simulink model "Ejercicio_2b"  (R2013a)
settings: Solver=ode45  StartTime=0.0  StopTime=40.0  RelTol=1e-3
InitFcn:
  | G1n=1;
  | G2n=1;
  | G3n=1;
  | G4n=1;
  | G5n=5;
  | G6n=1;
  | G7n=3;
  | G8n=1;
  | G1d=[1 7];
  | G2d=[1 2 3];
  | G3d=[1 4];
  | G4d=[1 0];
  | G5d=[1 7];
  | G6d=[1 5 10];
  | G7d=[1 2];
  | G8d=[1 6];
StartFcn:
  | G1n=1;
  | G2n=1;
  | G3n=1;
  | G4n=1;
  | G5n=5;
  | G6n=1;
  | G7n=3;
  | G8n=1;
  | G1d=[1 7];
  | G2d=[1 2 3];
  | G3d=[1 4];
  | G4d=[1 0];
  | G5d=[1 7];
  | G6d=[1 5 10];
  | G7d=[1 2];
  | G8d=[1 6];
settings Model: Creator=LuisFernando  LastModifiedBy=LuisFernando

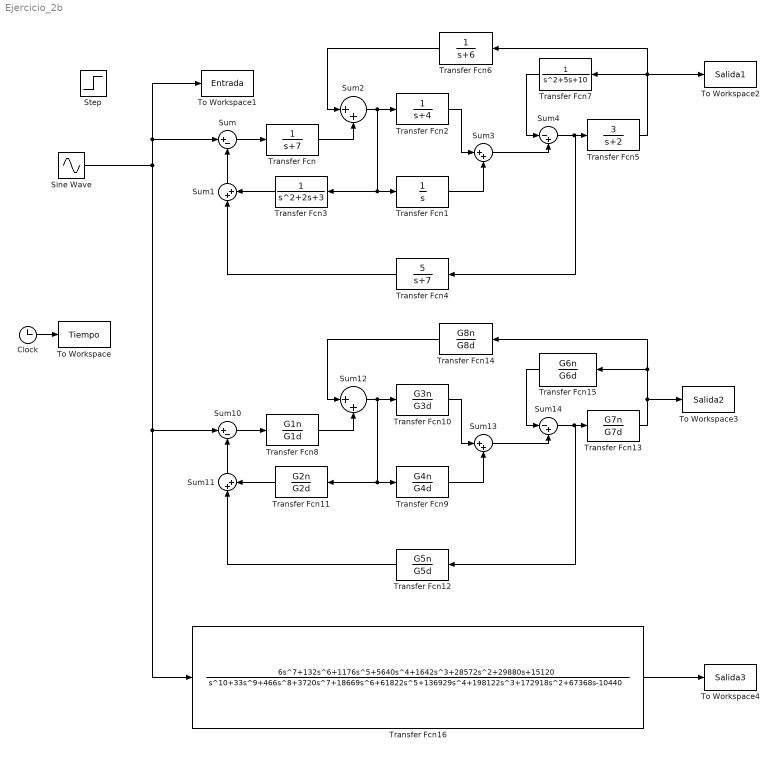
== system Ejercicio_2b ==
  Clock : Clock
  Sine Wave : Sin  Frequency=15  SampleTime=0
  Step : Step  SampleTime=0
  Sum : Sum  Inputs=|+-
  Sum{1..3,11..13} (6 alike) : Sum  Inputs=|++
  Sum10 : Sum  Inputs=|+-
  Sum14 : Sum  Inputs=|-+
  Sum4 : Sum  Inputs=|-+
  To Workspace : ToWorkspace  VariableName=Tiempo  SampleTime=-1
  To Workspace1 : ToWorkspace  VariableName=Entrada  SampleTime=-1
  To Workspace2 : ToWorkspace  VariableName=Salida1  SampleTime=-1
  To Workspace3 : ToWorkspace  VariableName=Salida2  SampleTime=-1
  To Workspace4 : ToWorkspace  VariableName=Salida3  SampleTime=-1
  Transfer Fcn : TransferFcn  Denominator=[1 7]
  Transfer Fcn1 : TransferFcn  Denominator=[1 0]
  Transfer Fcn10 : TransferFcn  Numerator=G3n  Denominator=G3d
  Transfer Fcn11 : TransferFcn  Numerator=G2n  Denominator=G2d
  Transfer Fcn12 : TransferFcn  Numerator=G5n  Denominator=G5d
  Transfer Fcn13 : TransferFcn  Numerator=G7n  Denominator=G7d
  Transfer Fcn14 : TransferFcn  Numerator=G8n  Denominator=G8d
  Transfer Fcn15 : TransferFcn  Numerator=G6n  Denominator=G6d
  Transfer Fcn16 : TransferFcn  Numerator=[6,132,1176,5640,1642,28572,29880,15120]  Denominator=[1,33,466,3720,18669,61822,136929,198122,172918,67368,-10440]
  Transfer Fcn2 : TransferFcn  Denominator=[1 4]
  Transfer Fcn3 : TransferFcn  Denominator=[1 2 3]
  Transfer Fcn4 : TransferFcn  Numerator=[5]  Denominator=[1 7]
  Transfer Fcn5 : TransferFcn  Numerator=[3]  Denominator=[1 2]
  Transfer Fcn6 : TransferFcn  Denominator=[1 6]
  Transfer Fcn7 : TransferFcn  Denominator=[1 5 10]
  Transfer Fcn8 : TransferFcn  Numerator=G1n  Denominator=G1d
  Transfer Fcn9 : TransferFcn  Numerator=G4n  Denominator=G4d
  wires:
  Transfer Fcn6/1 -> Sum2/1
  Transfer Fcn/1 -> Sum2/2
  Sum/1 -> Transfer Fcn/1
  Sum1/1 -> Sum/2
  Transfer Fcn3/1 -> Sum1/2
  Transfer Fcn4/1 -> Sum1/1
  Transfer Fcn2/1 -> Sum3/1
  Transfer Fcn1/1 -> Sum3/2
  Sum3/1 -> Sum4/2
  Transfer Fcn7/1 -> Sum4/1
  Sum4/1 -> Transfer Fcn4/1, Transfer Fcn5/1
  Transfer Fcn5/1 -> To Workspace2/1, Transfer Fcn6/1, Transfer Fcn7/1
  Sum2/1 -> Transfer Fcn2/1, Transfer Fcn1/1, Transfer Fcn3/1
  Transfer Fcn14/1 -> Sum12/1
  Transfer Fcn8/1 -> Sum12/2
  Sum10/1 -> Transfer Fcn8/1
  Sum11/1 -> Sum10/2
  Transfer Fcn11/1 -> Sum11/2
  Transfer Fcn12/1 -> Sum11/1
  Transfer Fcn10/1 -> Sum13/1
  Transfer Fcn9/1 -> Sum13/2
  Sum13/1 -> Sum14/2
  Transfer Fcn15/1 -> Sum14/1
  Sum14/1 -> Transfer Fcn12/1, Transfer Fcn13/1
  Sum12/1 -> Transfer Fcn10/1, Transfer Fcn9/1, Transfer Fcn11/1
  Clock/1 -> To Workspace/1
  Transfer Fcn13/1 -> Transfer Fcn14/1, Transfer Fcn15/1, To Workspace3/1
  Transfer Fcn16/1 -> To Workspace4/1
  Sine Wave/1 -> To Workspace1/1, Sum/1, Transfer Fcn16/1, Sum10/1
